simulink model "simPodC"  (R2024b)
settings: Solver=VariableStepAuto  StartTime=0.0  StopTime=10.0  RelTol=1e-3
values from neighbouring files (symbols this model uses):
  B = 20    [mFilePodA.m]    (also in mFilePodB.m)
  g = 9.81    [mFilePodA.m]    (also in mFilePodB.m)
  k = 200    [mFilePodA.m]    (also in mFilePodB.m)
  M = 10    [mFilePodA.m]    (also in mFilePodB.m)
settings Model: Creator=Ishak  LastModifiedBy=Ishak

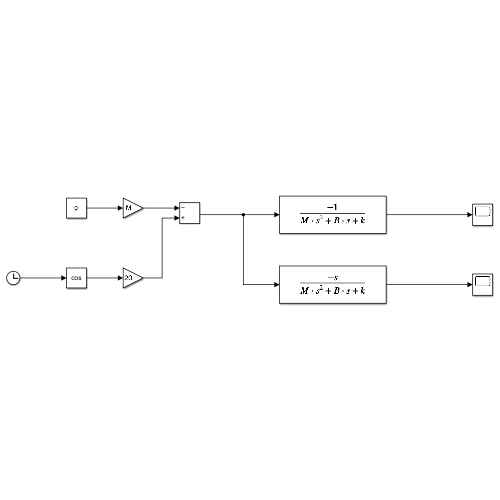
[thumbnail: Simulink's stored preview of the top-level diagram]
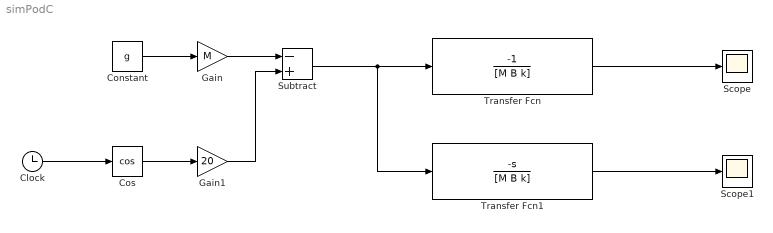
== system simPodC ==
  Clock : Clock
  Constant : Constant  Value=g
  Cos : Trigonometry  Operator=cos
  Gain : Gain  Gain=M
  Gain1 : Gain  Gain=20
  Scope : Scope
  Scope1 : Scope
  Subtract : Sum  Inputs=-+
  Transfer Fcn : TransferFcn  Numerator=[-1]  Denominator=[M B k]
  Transfer Fcn1 : TransferFcn  Numerator=[-1 0]  Denominator=[M B k]
  wires:
  Constant/1 -> Gain/1
  Gain/1 -> Subtract/1
  Clock/1 -> Cos/1
  Gain1/1 -> Subtract/2
  Cos/1 -> Gain1/1
  Subtract/1 -> Transfer Fcn1/1, Transfer Fcn/1
  Transfer Fcn/1 -> Scope/1
  Transfer Fcn1/1 -> Scope1/1
